simulink model "LNB_ET_Gr3_Simulink"  (R2023a)
settings: Solver=ode4  StartTime=0.0  StopTime=500  FixedStep=1/500  RelTol=1e-3
values from neighbouring files (symbols this model uses):
  A = [ -1/Ty           0               0                 0                 0 ... (first row only)    [LNB_ET_Gr3_Matlab.m]
  A_h = A    [LNB_ET_Gr3_Matlab.m]
  Ah = A    [LNB_ET_Gr3_Matlab.m]
  B = [ Ky/Ty ... (first row only)    [LNB_ET_Gr3_Matlab.m]
  B_h = [B,[0;0;0;0;0],[0;0;0;0;0]]    [LNB_ET_Gr3_Matlab.m]
  Bh = B    [LNB_ET_Gr3_Matlab.m]
  C = [0 0 0 0 KR]    [LNB_ET_Gr3_Matlab.m]
  C_h = C    [LNB_ET_Gr3_Matlab.m]
  C_R = [0 0 1 0 0]    [LNB_ET_Gr3_Matlab.m]
  Ch = C    [LNB_ET_Gr3_Matlab.m]
  D = [0]    [LNB_ET_Gr3_Matlab.m]
  E = [0        0 ... (first row only)    [LNB_ET_Gr3_Matlab.m]
  KD = 20    [LNB_ET_Gr3_Matlab.m]
  Kh = 1000    [LNB_ET_Gr3_Matlab.m]
  Kpv = 1    [LNB_ET_Gr3_Matlab.m]
  KR = 1/100    (= 0.01)    [LNB_ET_Gr3_Matlab.m]
  KRt = 1    [LNB_ET_Gr3_Matlab.m]
  KW = 1    [LNB_ET_Gr3_Matlab.m]
  Ky = 3/40    (= 0.075)    [LNB_ET_Gr3_Matlab.m]
  Kz = 2/100    (= 0.02)    [LNB_ET_Gr3_Matlab.m]
  L2 = L2T'    [LNB_ET_Gr3_Matlab.m]
  L_K = L_Kalman'    [LNB_ET_Gr3_Matlab.m]
  L_luen = L_luen_T'    [LNB_ET_Gr3_Matlab.m]
  LKalman = LKalmanT'    [LNB_ET_Gr3_Matlab.m]
  M = (C*(B*R_place-A)^(-1)*B)^(-1)    [LNB_ET_Gr3_Matlab.m]
  M1 = (C_R*(B*R_place_opt1-A)^(-1)*B)^(-1)    [LNB_ET_Gr3_Matlab.m]
  M2 = (C_R*(B*R_place_opt2-A)^(-1)*B)^(-1)    [LNB_ET_Gr3_Matlab.m]
  M3 = (C_R*(B*R_place_opt3-A)^(-1)*B)^(-1)    [LNB_ET_Gr3_Matlab.m]
  M4 = (C_R*(B*R_place_opt4-A)^(-1)*B)^(-1)    [LNB_ET_Gr3_Matlab.m]
  M_K = ML    [LNB_ET_Gr3_Matlab.m]
  M_lqr1 = (C_R*(B*R_place_lqr1-A)^(-1)*B)^(-1)    [LNB_ET_Gr3_Matlab.m]
  M_lqr2 = (C_R*(B*R_place_lqr2-A)^(-1)*B)^(-1)    [LNB_ET_Gr3_Matlab.m]
  M_lqr3 = (C_R*(B*R_place_lqr3-A)^(-1)*B)^(-1)    [LNB_ET_Gr3_Matlab.m]
  M_lqr4 = (C_R*(B*R_place_lqr4-A)^(-1)*B)^(-1)    [LNB_ET_Gr3_Matlab.m]
  ML = (C*(B*RL-A)^(-1)*B)^(-1)    [LNB_ET_Gr3_Matlab.m]
  R_I = -R_place_PI(:,6)    [LNB_ET_Gr3_Matlab.m]
  R_K = RL    [LNB_ET_Gr3_Matlab.m]
  R_p = -(C_R*Api^-1*Bpi)^-1    [LNB_ET_Gr3_Matlab.m]
  R_place = place(A,B,P_set)    [LNB_ET_Gr3_Matlab.m]
  R_place_lqr1 = lqr(A,B,Q1,R)    [LNB_ET_Gr3_Matlab.m]
  R_place_lqr2 = lqr(A,B,Q2,R)    [LNB_ET_Gr3_Matlab.m]
  R_place_lqr3 = lqr(A,B,Q3,R)    [LNB_ET_Gr3_Matlab.m]
  R_place_lqr4 = lqr(A,B,Q4,R)    [LNB_ET_Gr3_Matlab.m]
  R_place_opt1 = place(A,B,P_set_min1)    [LNB_ET_Gr3_Matlab.m]
  R_place_opt2 = place(A,B,P_set_min2)    [LNB_ET_Gr3_Matlab.m]
  R_place_opt3 = place(A,B,P_set_min3)    [LNB_ET_Gr3_Matlab.m]
  R_place_opt4 = place(A,B,P_set_min4)    [LNB_ET_Gr3_Matlab.m]
  R_x = R_place_PI(:,1:5)-R_p*C_R    [LNB_ET_Gr3_Matlab.m]
  Ri_F = -R_PI_F(1,6)    [LNB_ET_Gr3_Matlab.m]
  RL = place(A,B,P_set_L1)    [LNB_ET_Gr3_Matlab.m]
  Rp_F = -(C_R*A^(-1)*B(:,1))^(-1)    [LNB_ET_Gr3_Matlab.m]
  Rx_F = R_PI_F(1,1:5)-Rp_F*C_R    [LNB_ET_Gr3_Matlab.m]
  TD = 1/2    (= 0.5)    [LNB_ET_Gr3_Matlab.m]
  TRt = 1/250    (= 0.004)    [LNB_ET_Gr3_Matlab.m]
  TW1 = 20    [LNB_ET_Gr3_Matlab.m]
  TW2 = 50    [LNB_ET_Gr3_Matlab.m]
  Ty = 1/100    (= 0.01)    [LNB_ET_Gr3_Matlab.m]
  xs = [0;0;0;0;0]    [LNB_ET_Gr3_Matlab.m]
  Z = ((B')*B)^(-1)*(B')*E    [LNB_ET_Gr3_Matlab.m]
libraries: simulink x2
settings Model: Creator=bahad  LastModifiedBy=ziqii

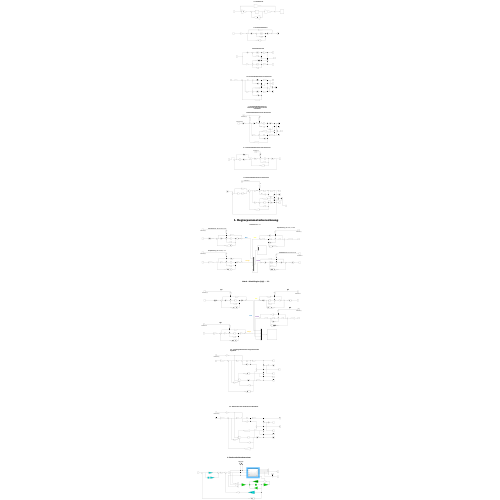
[thumbnail: Simulink's stored preview of the top-level diagram]
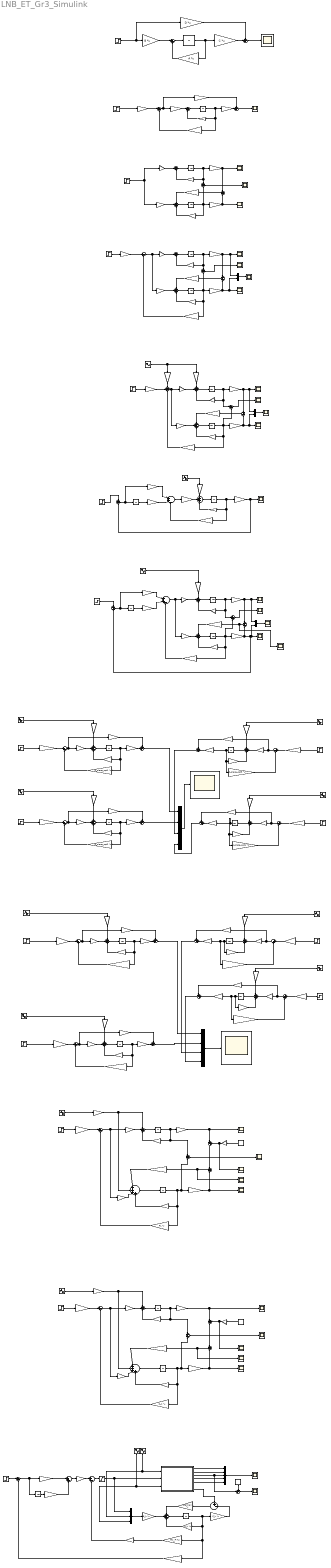
== system LNB_ET_Gr3_Simulink ==
  note: STÖRGRÖßEN (x2)
  note: X.
  note: ZUSTANDSBEOBACHTER
  note: RI
  note: Rp
  note: E*z
  note: STÖRGRÖßEN (x2)
  note: 1. SYSTEMANALYSE
  note: 3- Reglerparameterberechnung
  note: 2.1.1 ZUSTANDSREGELKREIS
  note: STÖRGRÖßEN (x2)
  note: FÜHRUNGSGRÖßE (x1)
  note: Blau
  note: E*z
  note: B*u
  note: STÖRGRÖßEN (x2)
  note: 2.1.3 ZUSTANDSRAUMREGELUNG MIT BEOBACHTER UNTER BEACHTUNG DER STÖRGRÖßEN
  note: B*u
  note: Polplatzierung - D = 0.9, T = 5
  note: STÖRGRÖßEN (x2)
  note: A*X
  note: STÖRGRÖßEN (x2)
  note: Q4
  note: Q3
  note: X
  note: Polplatzierung - D = 0.72, T = 5
  note: PI - ZUSTANDSGRÖßENREGELUNG OHNE BEOBACHTER
  note: Q1
  note: X
  note: STÖRGRÖßEN (x2)
  note: 2.1.2 ZUSTANDSRAUMREGELUNG MIT BEOBACHTER
  note: Matrix - Ricatti Regler (LQR) - 3.2
  note: STÖRGRÖßEN (x2)
  note: STÖRGRÖßEN (x2)
  note: STÖRGRÖßENKOMPENSATION MIT BEOBACHTER
  note: Q2
  note: STÖRGRÖßEN (x2)
  note: STÖRGRÖßEN (x2)
  note: STÖRGRÖßEN (x2)
  note: Polplatzierung - 3.1
  note: Polplatzierung - D = 0.72, T = 9.5
  note: Orange
  note: STÖRGRÖßEN (x2)
  note: Gelb
  note: A*X
  note: Violett
  note: X.
  note: Orange
  note: Blau
  note: 3.3 - Luenburger Beobachter mit geschlossenem Regelkreis
  note: Violett
  note: Rp
  note: 3.4 - Kalman Bucy mit geschlossenem Regelkreis
  note: RI
  note: Gelb
  note: PI - ZUSTANDSGRÖßENREGELUNG MIT BEOBACHTER
  note: Polplatzierung - D = 0.9, T = 9.5
  note: uY
  note: Nichtlineares Systemmodell
  note: Störgrößen
  note: Pv
  note: m.w
  note: 4. Reglerverhaltensbewertung
  Band-Limited White Noise : simulink/Sources/Band-Limited White Noise  Cov=[0.003]  Ts=0.1  seed=[23341]
  Band-Limited White Noise1 : simulink/Sources/Band-Limited White Noise  Cov=[0.003]  Ts=0.1  seed=[23341]
  Constant : Constant  Value=50
  Gain{,4,10,17,27,31,45,48,53,70,77,84,87,98,105,112,118} (17 alike) : Gain  Gain=B  Multiplication=Matrix(K*u)
  Gain{1,6,12,19,33,55,115,126} (8 alike) : Gain  Gain=C  Multiplication=Matrix(K*u)
  Gain{30,44,47,50,52,72,79,86,89,100,107,114,125} (13 alike) : Gain  Gain=E  Multiplication=Matrix(K*u)
  Gain{43,62..63,73,80,90..91,101,108,135} (10 alike) : Gain  Gain=C_R  Multiplication=Matrix(K*u)
  Gain102 : Gain  Gain=M_lqr3  Multiplication=Matrix(K*u)
  Gain103 : Gain  Gain=R_place_lqr3  Multiplication=Matrix(K*u)
  Gain{2,9,67,69,76,83,95,97,104,111} (10 alike) : Gain  Gain=D  Multiplication=Matrix(K*u)
  Gain{3,5,11,18,28,32,46,49,54,71,78,85,88,99,106,113,124} (17 alike) : Gain  Gain=A  Multiplication=Matrix(K*u)
  Gain109 : Gain  Gain=M_lqr4  Multiplication=Matrix(K*u)
  Gain110 : Gain  Gain=R_place_lqr4  Multiplication=Matrix(K*u)
  Gain116 : Gain  Gain=ML  Multiplication=Matrix(K*u)
  Gain117 : Gain  Gain=0
  Gain{14,21,36,57,119,129} (6 alike) : Gain  Gain=Ah  Multiplication=Matrix(K*u)
  Gain120 : Gain  Gain=RL  Multiplication=Matrix(K*u)
  Gain{15,22,37,58,121,131} (6 alike) : Gain  Gain=Ch  Multiplication=Matrix(K*u)
  Gain122 : Gain  Gain=L2  Multiplication=Matrix(K*u)
  Gain{13,20,35,56,123,133} (6 alike) : Gain  Gain=Bh  Multiplication=Matrix(K*u)
  Gain127 : Gain  Gain=M_K  Multiplication=Matrix(K*u)
  Gain128 : Gain
  Gain130 : Gain  Gain=R_K  Multiplication=Matrix(K*u)
  Gain132 : Gain  Gain=L_K  Multiplication=Matrix(K*u)
  Gain134 : Gain  Gain=Ri_F  Multiplication=Matrix(K*u)
  Gain136 : Gain
  Gain137 : Gain  Gain=Rp_F  Multiplication=Matrix(K*u)
  Gain138 : Gain  Gain=Rx_F  Multiplication=Matrix(K*u)
  Gain139 : Gain  Gain=LKalman  Multiplication=Matrix(K*u)
  Gain140 : Gain  Gain=B_h  Multiplication=Matrix(K*u)
  Gain141 : Gain  Gain=A_h  Multiplication=Matrix(K*u)
  Gain142 : Gain  Gain=C_h  Multiplication=Matrix(K*u)
  Gain{16,23,38,59} (4 alike) : Gain  Gain=L_luen  Multiplication=Matrix(K*u)
  Gain24 : Gain  Gain=R_place  Multiplication=Matrix(K*u)
  Gain25 : Gain  Gain=M  Multiplication=Matrix(K*u)
  Gain26 : Gain  Gain=Z  Multiplication=Matrix(K*u)
  Gain29 : Gain  Gain=0.5
  Gain34 : Gain  Gain=R_I  Multiplication=Matrix(K*u)
  Gain39 : Gain  Gain=M  Multiplication=Matrix(K*u)
  Gain40 : Gain  Gain=R_place  Multiplication=Matrix(K*u)
  Gain41 : Gain  Gain=R_x  Multiplication=Matrix(K*u)
  Gain42 : Gain  Gain=R_p  Multiplication=Matrix(K*u)
  Gain51 : Gain  Gain=R_I  Multiplication=Matrix(K*u)
  Gain60 : Gain  Gain=R_p  Multiplication=Matrix(K*u)
  Gain61 : Gain  Gain=R_x  Multiplication=Matrix(K*u)
  Gain64 : Gain  Gain=M4  Multiplication=Matrix(K*u)
  Gain65 : Gain  Gain=M1  Multiplication=Matrix(K*u)
  Gain66 : Gain  Gain=R_place_opt1  Multiplication=Matrix(K*u)
  Gain68 : Gain  Gain=R_place_opt4  Multiplication=Matrix(K*u)
  Gain7 : Gain  Gain=M  Multiplication=Matrix(K*u)
  Gain74 : Gain  Gain=M2  Multiplication=Matrix(K*u)
  Gain75 : Gain  Gain=R_place_opt2  Multiplication=Matrix(K*u)
  Gain8 : Gain  Gain=R_place  Multiplication=Matrix(K*u)
  Gain81 : Gain  Gain=M3  Multiplication=Matrix(K*u)
  Gain82 : Gain  Gain=R_place_opt3  Multiplication=Matrix(K*u)
  Gain92 : Gain  Gain=M_lqr2  Multiplication=Matrix(K*u)
  Gain93 : Gain  Gain=M_lqr1  Multiplication=Matrix(K*u)
  Gain94 : Gain  Gain=R_place_lqr1  Multiplication=Matrix(K*u)
  Gain96 : Gain  Gain=R_place_lqr2  Multiplication=Matrix(K*u)
  Integrator{,1,3,5..6,8..11,13..21,23,26} (20 alike) : Integrator
  Integrator{2,4,7,12} (4 alike) : Integrator  InitialCondition=[1 2 3 4 5]
  Integrator22 : Integrator  InitialCondition=[1 1 1 1 1]
  Integrator24 : Integrator  InitialCondition=[1 1 1 1 1]
  Integrator25 : Integrator  InitialCondition=xs
  Mux : Mux  Inputs=2
  Mux1 : Mux  Inputs=2
  Mux2 : Mux  Inputs=2
  Mux3 : Mux
  Mux4 : Mux  Inputs=3
  Mux5 : Mux  Inputs=5
  Mux7 : Mux
  Saturation : Saturate  UpperLimit=5  LowerLimit=-5
  Scope{,1..32} (33 alike) : Scope
  Sine Wave{,1..11,13} (13 alike) : Sin  Amplitude=[1 10]  Frequency=[2*pi*(10^-2) 2*pi*(1/300)]  SampleTime=0
  Sine Wave12 : Sin  Amplitude=10  Frequency=2*pi*(1/300)  SampleTime=0
  Sine Wave14 : Sin  Frequency=2*pi*(10^-2)  SampleTime=0
  Step{1..17,19} (18 alike) : Step  Time=10  Before=20  After=45  SampleTime=0
  Subsystem2 : Subsystem
  Sum{,3,23,32,35,38,41,44,47,50,69} (11 alike) : Sum  Inputs=++|
  Sum{1..2,5,9,53,59,64} (7 alike) : Sum  Inputs=|++
  Sum{6,10,15..16,21..22,24,26,29,34,37,40,42,46,49,52,58,67} (18 alike) : Sum  Inputs=+++
  Sum{7..8,11..12,17..18,27..28,56..57,62..63} (12 alike) : Sum  Inputs=+-
  Sum{4,13..14,25,31,33,36,39,43,45,48,51,54,60,65..66} (16 alike) : Sum  Inputs=|+-
  Sum19 : Sum  Inputs=-+-
  Sum20 : Sum  Inputs=|++-
  Sum30 : Sum  Inputs=|++-
  Sum55 : Sum  Inputs=|++++
  Sum61 : Sum  Inputs=|++++
  Sum68 : Sum  Inputs=+-|
  wires:
  Gain48/1 -> Sum24/2
  Gain76/1 -> Sum35/1
  Sum25/1 -> Scope16/1
  Sine Wave7/1 -> Gain72/1
  Step5/1 -> Sum18/1
  Step10/1 -> Gain74/1
  Gain79/1 -> Sum37/1
  Gain20/1 -> Sum10/2
  Sum17/1 -> Gain38/1
  Gain99/1 -> Sum46/3
  Sum36/1 -> Gain76/1, Gain70/1
  Gain56/1 -> Sum26/2
  Gain49/1 -> Sum24/3
  Gain66/1 -> Sum31/2
  Gain64/1 -> Sum33/1
  Gain121/1 -> Scope20/1, Sum57/2
  Gain123/1 -> Sum55/3
  Sum58/1 -> Integrator23/1
  Gain69/1 -> Sum32/1
  Sum52/1 -> Integrator21/1
  Sum47/1 -> Mux7/3
  Sum45/1 -> Gain97/1, Gain87/1
  Integrator24/1 -> Gain131/1, Sum62/2, Gain130/1, Gain129/1
  Gain12/1 -> Scope3/1, Sum7/1
  Gain40/1 -> Sum19/3
  Gain118/1 -> Sum58/2
  Sum19/1 -> Gain35/1, Gain31/1
  Sum63/1 -> Scope26/1, Gain132/1
  Gain33/1 -> Mux1/1, Scope9/1, Sum17/1
  Gain82/1 -> Sum39/2
  Gain67/1 -> Sum23/1
  Integrator10/1 -> Gain46/1, Gain66/1, Gain63/1
  Integrator9/1 -> Gain34/1
  Integrator5/1 -> Gain22/1, Gain24/1, Gain21/1, Sum12/2
  Sum54/1 -> Gain123/1, Gain112/1
  Gain89/1 -> Sum42/1
  Integrator4/1 -> Gain19/1, Gain18/1, Sum12/1
  Gain23/1 -> Sum10/1
  Gain21/1 -> Sum10/3
  Integrator17/1 -> Gain88/1, Gain96/1, Gain90/1
  Sum34/1 -> Integrator15/1
  Gain119/1 -> Sum55/4
  Gain117/1 -> Sum53/2, Scope24/1
  Gain96/1 -> Sum45/2
  Sine Wave13/1 -> Gain125/1
  Gain2/1 -> Sum/1
  Gain17/1 -> Sum9/1
  Sum59/1 -> Sum63/1
  Integrator21/1 -> Sum56/1, Gain113/1, Gain115/1
  Gain73/1 -> Sum35/2
  Mux3/1 -> Scope19/1
  Mux2/1 -> Scope17/1
  Sine Wave8/1 -> Gain79/1
  Sum14/1 -> Scope11/1
  Step15/1 -> Gain102/1
  Integrator11/1 -> Gain49/1, Gain68/1, Gain62/1
  Sum38/1 -> Mux3/3
  Integrator16/1 -> Gain78/1, Gain82/1, Gain80/1
  Sine Wave5/1 -> Gain50/1
  Sum33/1 -> Gain69/1, Gain48/1
  Sum62/1 -> Scope28/1
  Gain59/1 -> Sum26/1
  Step8/1 -> Gain65/1
  Gain46/1 -> Sum22/3
  Gain65/1 -> Sum31/1
  Gain77/1 -> Sum37/2
  Gain50/1 -> Sum24/1
  Gain47/1 -> Sum22/1
  Sum31/1 -> Gain67/1, Gain45/1
  Sum3/1 -> Scope1/1
  Gain32/1 -> Sum21/3
  Gain57/1 -> Sum26/3
  Gain75/1 -> Sum36/2
  Gain62/1 -> Sum32/2
  Gain51/1 -> Sum30/2
  Gain111/1 -> Sum50/1
  Sum21/1 -> Integrator7/1
  Sum37/1 -> Integrator16/1
  Integrator18/1 -> Gain103/1, Gain101/1, Gain99/1
  Sum61/1 -> Integrator24/1
  Gain126/1 -> Sum59/1, Scope29/1
  Gain124/1 -> Sum58/3
  Gain18/1 -> Sum9/2
  Gain133/1 -> Sum61/3
  Sum48/1 -> Gain104/1, Gain98/1
  Gain132/1 -> Sum61/1
  Gain125/1 -> Sum61/2, Sum58/1
  Gain10/1 -> Sum5/1
  Gain39/1 -> Sum19/2
  Sum60/1 -> Gain133/1, Gain118/1
  Step12/1 -> Gain93/1
  Sum28/1 -> Gain60/1, Integrator14/1
  Gain130/1 -> Sum60/2
  Gain116/1 -> Sum54/1
  Sum10/1 -> Integrator5/1
  Gain127/1 -> Sum60/1
  Band-Limited White Noise/1 -> Gain117/1
  Integrator20/1 -> Gain110/1, Gain108/1, Gain106/1
  Integrator23/1 -> Sum62/1, Gain124/1, Gain126/1
  Gain122/1 -> Sum55/1
  Gain112/1 -> Sum52/2
  Gain114/1 -> Sum55/2, Sum52/1
  Integrator22/1 -> Gain121/1, Sum56/2, Gain120/1, Gain119/1
  Gain113/1 -> Sum52/3
  Gain120/1 -> Sum54/2
  Step17/1 -> Gain116/1
  Gain128/1 -> Sum59/2, Scope30/1
  Gain115/1 -> Sum53/1, Scope22/1
  Integrator7/1 -> Gain33/1, Sum14/1, Gain32/1
  Sum50/1 -> Mux7/4
  Gain105/1 -> Sum49/2
  Sum39/1 -> Gain83/1, Gain77/1
  Sine Wave11/1 -> Gain107/1
  Gain109/1 -> Sum51/1
  Gain106/1 -> Sum49/3
  Step16/1 -> Gain109/1
  Gain26/1 -> Sum19/1
  Gain95/1 -> Sum41/1
  Sum22/1 -> Integrator10/1
  Gain53/1 -> Sum29/2
  Gain63/1 -> Sum23/2
  Gain80/1 -> Sum38/2
  Gain94/1 -> Sum43/2
  Gain110/1 -> Sum51/2
  Gain34/1 -> Sum20/2
  Sum49/1 -> Integrator20/1
  Step3/1 -> Gain25/1
  Gain104/1 -> Sum47/1
  Gain85/1 -> Sum40/3
  Gain103/1 -> Sum48/2
  Sum30/1 -> Gain56/1, Gain53/1
  Gain87/1 -> Sum42/2
  Sine Wave9/1 -> Gain89/1
  Sine Wave6/1 -> Gain86/1
  Gain100/1 -> Sum46/1
  Gain98/1 -> Sum46/2
  Gain74/1 -> Sum36/1
  Gain84/1 -> Sum40/2
  Sum42/1 -> Integrator17/1
  Gain61/1 -> Sum30/3
  Mux7/1 -> Scope25/1
  Mux1/1 -> Scope12/1
  Step4/1 -> Gain39/1
  Integrator19/1 -> Gain85/1, Gain94/1, Gain91/1
  Sum16/1 -> Integrator8/1
  Step14/1 -> Gain92/1
  Sum24/1 -> Integrator11/1
  Sum40/1 -> Integrator19/1
  Gain92/1 -> Sum45/1
  Gain88/1 -> Sum42/3
  Sum26/1 -> Integrator13/1
  Gain78/1 -> Sum37/3
  Sum8/1 -> Scope4/1
  Sine Wave10/1 -> Gain100/1
  Sum53/1 -> Sum57/1
  Gain58/1 -> Scope15/1, Mux2/2, Sum28/2, Sum27/2
  Step6/1 -> Sum28/1
  Sum44/1 -> Mux7/2
  Gain60/1 -> Sum30/1
  Integrator13/1 -> Gain58/1, Sum25/2, Gain61/1, Gain57/1
  Gain44/1 -> Sum15/1
  Sum29/1 -> Integrator12/1
  Sum18/1 -> Gain42/1, Integrator9/1
  Sine Wave1/1 -> Gain44/1
  Sum20/1 -> Gain27/1
  Gain90/1 -> Sum44/2
  Gain30/1 -> Sum21/1
  Gain41/1 -> Sum20/3
  Integrator12/1 -> Gain55/1, Sum25/1, Gain54/1
  Sum27/1 -> Scope23/1, Gain59/1
  Gain81/1 -> Sum39/1
  Gain97/1 -> Sum44/1
  Gain108/1 -> Sum50/2
  Gain5/1 -> Sum2/2
  Mux/1 -> Scope8/1
  Sum6/1 -> Integrator3/1
  Sum/1 -> Scope/1
  Gain36/1 -> Sum16/3
  Sum32/1 -> Mux3/4
  Gain42/1 -> Sum20/1
  Sum15/1 -> Integrator6/1
  Integrator6/1 -> Gain41/1, Gain28/1, Gain43/1
  Step7/1 -> Gain2/1, Gain/1
  Gain38/1 -> Sum16/1
  Sine Wave/1 -> Gain30/1, Gain26/1
  Gain31/1 -> Sum21/2
  Gain27/1 -> Sum15/2
  Sum41/1 -> Mux7/1
  Gain131/1 -> Sum63/2, Scope27/1
  Sum43/1 -> Gain95/1, Gain84/1
  Gain55/1 -> Mux2/1, Scope18/1, Sum27/1
  Sum46/1 -> Integrator18/1
  Sum9/1 -> Integrator4/1
  Gain35/1 -> Sum16/2
  Gain37/1 -> Mux1/2, Scope10/1, Sum17/2
  Gain54/1 -> Sum29/3
  Gain25/1 -> Sum13/1
  Integrator3/1 -> Gain15/1, Gain14/1, Sum8/2
  Gain24/1 -> Sum13/2
  Sum11/1 -> Gain23/1
  Gain102/1 -> Sum48/1
  Sum7/1 -> Gain16/1
  Gain14/1 -> Sum6/3
  Gain6/1 -> Sum3/2
  Gain13/1 -> Sum6/2
  Gain15/1 -> Scope2/1, Sum7/2
  Step2/1 -> Gain13/1, Gain10/1
  Gain52/1 -> Sum29/1
  Integrator8/1 -> Gain37/1, Sum14/2, Gain40/1, Gain36/1
  Sum2/1 -> Integrator1/1
  Gain7/1 -> Sum4/1
  Gain86/1 -> Sum40/1
  Gain93/1 -> Sum43/1
  Sine Wave2/1 -> Gain114/1
  Integrator1/1 -> Gain8/1, Gain5/1, Gain6/1
  Gain8/1 -> Sum4/2
  Sum57/1 -> Scope14/1, Gain122/1
  Gain3/1 -> Sum1/2
  Step19/1 -> Gain127/1
  Gain1/1 -> Sum/2
  Gain4/1 -> Sum2/1
  Sum1/1 -> Integrator/1
  Gain91/1 -> Sum41/2
  Gain/1 -> Sum1/1
  Integrator/1 -> Gain3/1, Gain1/1
  Gain70/1 -> Sum34/2
  Gain28/1 -> Sum15/3
  Step9/1 -> Gain64/1
  Sum23/1 -> Mux3/1
  Gain16/1 -> Sum6/1
  Gain68/1 -> Sum33/2
  Gain71/1 -> Sum34/3
  Sum13/1 -> Gain20/1, Gain17/1
  Sine Wave3/1 -> Gain52/1
  Gain72/1 -> Sum34/1
  Gain129/1 -> Sum61/4
  Sine Wave4/1 -> Gain47/1
  Step1/1 -> Gain7/1
  Gain22/1 -> Mux/2, Scope5/1, Sum11/2
  Sum55/1 -> Integrator22/1
  Gain9/1 -> Sum3/1
  Integrator14/1 -> Gain51/1
  Sum56/1 -> Scope21/1
  Sum35/1 -> Mux3/2
  Sum5/1 -> Integrator2/1
  Gain101/1 -> Sum47/2
  Gain43/1 -> Sum18/2, Scope13/1
  Step13/1 -> Gain81/1
  Integrator2/1 -> Gain12/1, Gain11/1, Sum8/1
  Sum51/1 -> Gain111/1, Gain105/1
  Sum12/1 -> Scope7/1
  Sum4/1 -> Gain9/1, Gain4/1
  Gain45/1 -> Sum22/2
  Gain83/1 -> Sum38/1
  Band-Limited White Noise1/1 -> Gain128/1
  Integrator15/1 -> Gain71/1, Gain75/1, Gain73/1
  Gain19/1 -> Mux/1, Scope6/1, Sum11/1
  Gain11/1 -> Sum5/2
  Gain107/1 -> Sum49/1
  Integrator26/1 -> Gain134/1
  Step11/1 -> Sum66/1
  Sum65/1 -> Saturation/1
  Gain135/1 -> Sum66/2
  Subsystem2/4(T.aus) -> Mux5/4  "T.aus"
  Mux5/1 -> Scope31/1
  Gain142/1 -> Sum68/2
  Gain140/1 -> Sum67/2
  Subsystem2/2(m.D) -> Mux5/2  "m.D"
  Gain29/1 -> Sum65/1
  Mux4/1 -> Gain140/1
  Gain138/1 -> Gain136/1
  Gain137/1 -> Sum64/1
  Gain136/1 -> Sum65/2
  Sum68/1 -> Gain139/1
  Sum64/1 -> Gain29/1
  Gain139/1 -> Sum67/1
  Sine Wave12/1 -> Mux4/3, Subsystem2/3(z2 - m.w)
  Sine Wave14/1 -> Mux4/2, Subsystem2/1(z1 - Pv)
  Sum66/1 -> Integrator26/1, Gain137/1
  Sum69/1 -> Scope32/1
  Subsystem2/7(ym - Ut) -> Sum68/1
  Saturation/1 -> Mux4/1, Subsystem2/2(u - Uy)
  Constant/1 -> Sum69/1
  Integrator25/1 -> Gain142/1, Gain135/1, Gain138/1, Gain141/1
  Subsystem2/1(Py) -> Mux5/1  "Py"
  Subsystem2/3(x - Taus) -> Sum69/2, Mux5/3  "Taus"
  Gain134/1 -> Sum64/2
  Sum67/1 -> Integrator25/1
  Gain141/1 -> Sum67/3
  Subsystem2/5(Rt) -> Mux5/5  "Rt"

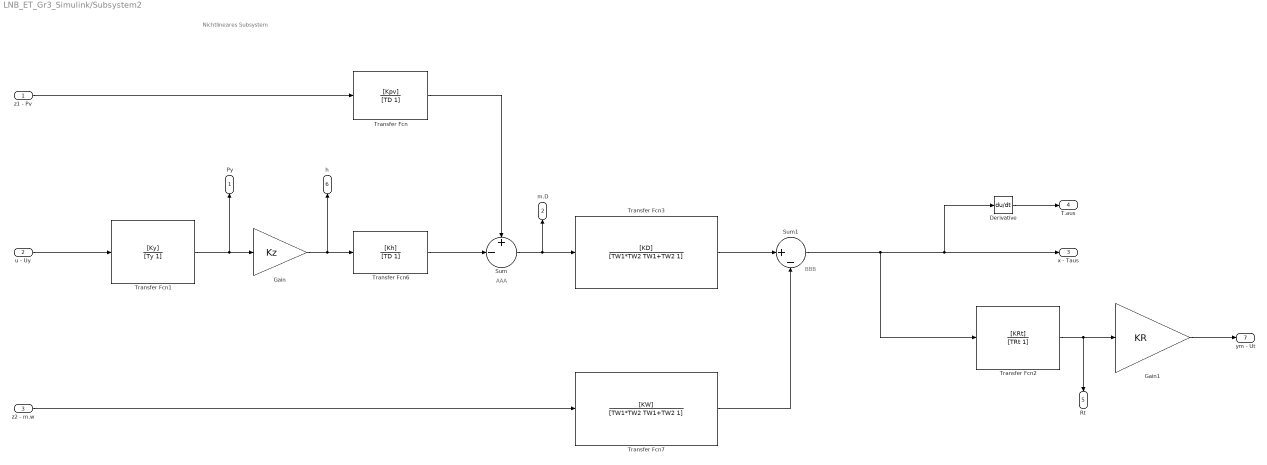
== system LNB_ET_Gr3_Simulink/Subsystem2 ==
  note: BBB
  note: AAA
  note: Nichtlineares Subsystem
  z1 - Pv : Inport
  u - Uy : Inport  Port=2
  z2 - m.w : Inport  Port=3
  Derivative : Derivative
  Gain : Gain  Gain=Kz
  Gain1 : Gain  Gain=KR
  Sum : Sum  Inputs=+-|
  Sum1 : Sum  Inputs=|+-
  Transfer Fcn : TransferFcn  Numerator=[Kpv]  Denominator=[TD 1]
  Transfer Fcn1 : TransferFcn  Numerator=[Ky]  Denominator=[Ty 1]
  Transfer Fcn2 : TransferFcn  Numerator=[KRt]  Denominator=[TRt 1]
  Transfer Fcn3 : TransferFcn  Numerator=[KD]  Denominator=[TW1*TW2 TW1+TW2 1]
  Transfer Fcn6 : TransferFcn  Numerator=[Kh]  Denominator=[TD 1]
  Transfer Fcn7 : TransferFcn  Numerator=[KW]  Denominator=[TW1*TW2 TW1+TW2 1]
  Py : Outport
  m.D : Outport  Port=2
  x - Taus : Outport  Port=3
  T.aus : Outport  Port=4
  Rt : Outport  Port=5
  h : Outport  Port=6
  ym - Ut : Outport  Port=7
  wires:
  Transfer Fcn1/1 -> Py/1, Gain/1
  Gain/1 -> h/1, Transfer Fcn6/1
  Transfer Fcn2/1 -> Rt/1, Gain1/1
  Gain1/1 -> ym - Ut/1
  z2 - m.w/1 -> Transfer Fcn7/1
  Transfer Fcn6/1 -> Sum/2
  Sum/1 -> m.D/1, Transfer Fcn3/1
  Transfer Fcn3/1 -> Sum1/1
  Transfer Fcn7/1 -> Sum1/2
  u - Uy/1 -> Transfer Fcn1/1
  Sum1/1 -> Transfer Fcn2/1, Derivative/1, x - Taus/1
  z1 - Pv/1 -> Transfer Fcn/1
  Transfer Fcn/1 -> Sum/1
  Derivative/1 -> T.aus/1
